simulink model "SimulinkSample"  (R2024b)
settings: Solver=VariableStepAuto  StartTime=0.0  StopTime=10.0  RelTol=1e-3
settings Model: Creator=saijaz  LastModifiedBy=saijaz

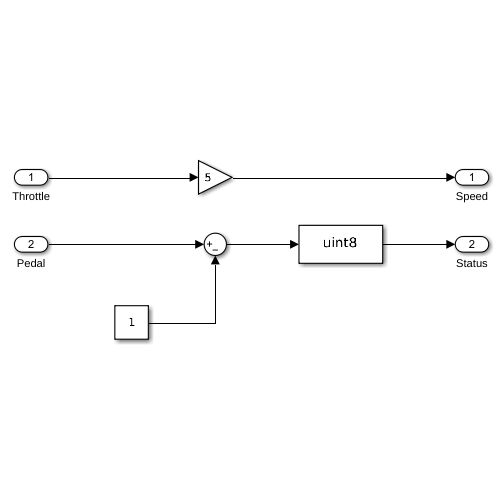
[thumbnail: Simulink's stored preview of the top-level diagram]
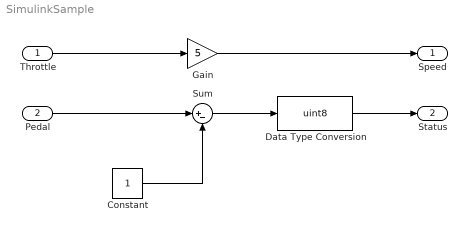
== system SimulinkSample ==
  Throttle : Inport  OutDataTypeStr=double
  Pedal : Inport  Port=2  OutDataTypeStr=double
  Constant : Constant  OutDataTypeStr=double
  Data Type Conversion : DataTypeConversion  OutDataTypeStr=uint8  SaturateOnIntegerOverflow=off  RndMeth=Floor
  Gain : Gain  Gain=5
  Sum : Sum  Inputs=|+-
  Speed : Outport
  Status : Outport  Port=2  OutDataTypeStr=uint8
  wires:
  Throttle/1 -> Gain/1
  Gain/1 -> Speed/1
  Constant/1 -> Sum/2
  Pedal/1 -> Sum/1
  Sum/1 -> Data Type Conversion/1
  Data Type Conversion/1 -> Status/1
